simulink library "aeroblk_lib_HL20"  (Simulink 6.0)
settings: Solver=ode45  SolverMode=SingleTasking  StartTime=0.0  StopTime=10.0  RelTol=1e-3
values from neighbouring files (symbols this model uses):
  a_matrix = [-0.028840208852 -0.0156596305643 -0.0560912779756 -0.0863202941854 0.0209519994416 0.0112571762889 23.9049039727 0 2.90446405277 0 -10.5841662935 0 ... (11560 elements, 17x17x8x5)]    [aeroblk_HL20_autopilot_gains.mat]
  A_matrix = [-0.028840208852 -0.0156596305643 -0.0560912779756 -0.0863202941854 0.0209519994416 0.0112571762889 0 0 0 0 0 0 ... (11560 elements, 17x17x8x5)]    [aeroblk_HL20_autopilot_gains.mat]
  alpha_vec_Cn0 = [-10 -5 0 5 10 15 20 25 30]    [aeroblk_init_HL20.m]
  b_matrix = [-0.0157218860845 -0.283968320777 0.321370128412 0.271058535159 0.0185568065093 -0.00784369239396 -0.320886300542 1.82463546416 -0.0471251877299 0.142152392032 -0.0609086167769 0.505612659091 ... (2040 elements, 17x3x8x5)]    [aeroblk_HL20_autopilot_gains.mat]
  B_matrix = [0 0 0 0 0 0 4 0 0 0 0 0 ... (2040 elements, 17x3x8x5)]    [aeroblk_HL20_autopilot_gains.mat]
  b_ref = 13.89/m2ft    (= 4.23367186452)    [aeroblk_init_HL20.m]
  beta_vec_Cn0 = [0 2 5 10]    [aeroblk_init_HL20.m]
  c_matrix = [-5.97622599319 -0.726116013193 2.64604157338 -40.7494939461 11.661494324 21.0342779763 20.6745716213 -19.9416021106 -13.12545371 926.002157715 -187.969629212 -231.434488107 ... (2040 elements, 3x17x8x5)]    [aeroblk_HL20_autopilot_gains.mat]
  C_matrix = [0 0 0 0 0 0 0 0 0 -58.994812472 0 0 ... (2040 elements, 3x17x8x5)]    [aeroblk_HL20_autopilot_gains.mat]
  Clbeta = -0.00787    [aeroblk_init_HL20.m]
  Cm0 = reshape(temp(:,2),length(beta_vec_0),length(alpha_vec_0))    [aeroblk_init_HL20.m]
  CX0 = -reshape(temp(:,3),length(beta_vec_0),length(alpha_vec_0))    [aeroblk_init_HL20.m]
  CYbeta = -0.01242    [aeroblk_init_HL20.m]
  CZ0 = -reshape(temp(:,1),length(beta_vec_0),length(alpha_vec_0))    [aeroblk_init_HL20.m]
  d_matrix = [0 0 0 0 0 0 0 0 0 0 0 0 ... (360 elements, 3x3x8x5)]    [aeroblk_HL20_autopilot_gains.mat]
  d_ref = 0.75/m2ft    (= 0.228599992685)    [aeroblk_guid_dat.m]    (also in aeroblk_init_HL20.m = 8.60755172456)
  F_matrix = [5.97622599319 0.726116013193 -2.64604157338 40.7494939461 -11.661494324 -21.0342779763 -20.6745716213 19.9416021106 13.12545371 -926.002157715 187.969629212 231.434488107 ... (2040 elements, 3x17x8x5)]    [aeroblk_HL20_autopilot_gains.mat]
  H_matrix = [-0.0157218860845 -0.283968320777 0.321370128412 0.271058535159 0.0185568065093 -0.00784369239396 -0.320886300542 1.82463546416 -0.0471251877299 0.142152392032 -0.0609086167769 0.505612659091 ... (2040 elements, 17x3x8x5)]    [aeroblk_HL20_autopilot_gains.mat]
  mass = 13.98/Kg2slug    (= 204.022661401)    [aeroblk_guid_dat.m]    (also in aeroblk_init_HL20.m = 11738.9844962)
  x_cg = 0.575*len_veh    (= 4.78635044684)    [aeroblk_init_HL20.m]
  x_ref = 0.54*len_veh    (= 4.49500737616)    [aeroblk_init_HL20.m]
undefined symbols (not defined in the file or in its folder): F, Light, MIL
libraries: simulink x60, aerolibconvert x4, aerolibschedule x4, aerolibasang x3, aerolibwind2 x3, aeroblk_lib_HL20 x1, aerolib6dof2 x1, aerolibatmos2 x1, aerolibgravity2 x1, aerolibadyn x1
(part 1 of 2)
settings Model: Creator=The MathWorks Inc.  LastModifiedBy=batserve  ExtModeAutoUpdateStatusClock=off
settings OptimizationCC: BooleanDataType=off
settings DebuggingCC: CheckExecutionContextPreStartOutputMsg=on  CheckExecutionContextRuntimeOutputMsg=on  SolverPrmCheckMsg=none
settings HardwareCC: TargetUnknown=on

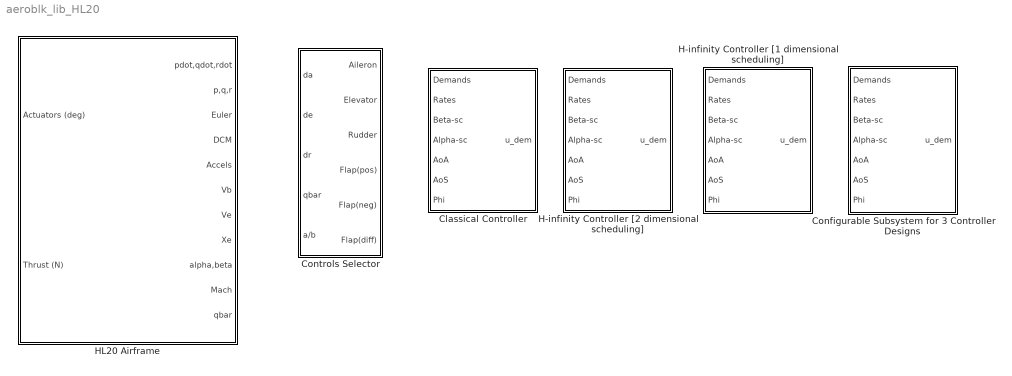
== system aeroblk_lib_HL20 ==
  Classical Controller : Subsystem  PropExecContextAcrossSSBoundary=on
  Configurable Subsystem for 3 Controller Designs : Subsystem  BlockChoice=Classical Controller  PropExecContextAcrossSSBoundary=on
      settings: TemplateBlock=self  MemberBlocks=Classical Controller,H-infinity Controller [1 dimensional scheduling],H-infinity Controller [2 dimensional scheduling]
  Controls Selector : Subsystem  PropExecContextAcrossSSBoundary=on
  H-infinity Controller [1 dimensional scheduling] : Subsystem  PropExecContextAcrossSSBoundary=on
  H-infinity Controller [2 dimensional scheduling] : Subsystem  PropExecContextAcrossSSBoundary=on
  HL20 Airframe : Subsystem  PropExecContextAcrossSSBoundary=on
      mask Display: image(imread('aeroblk_HL20pic.jpg','jpg'))

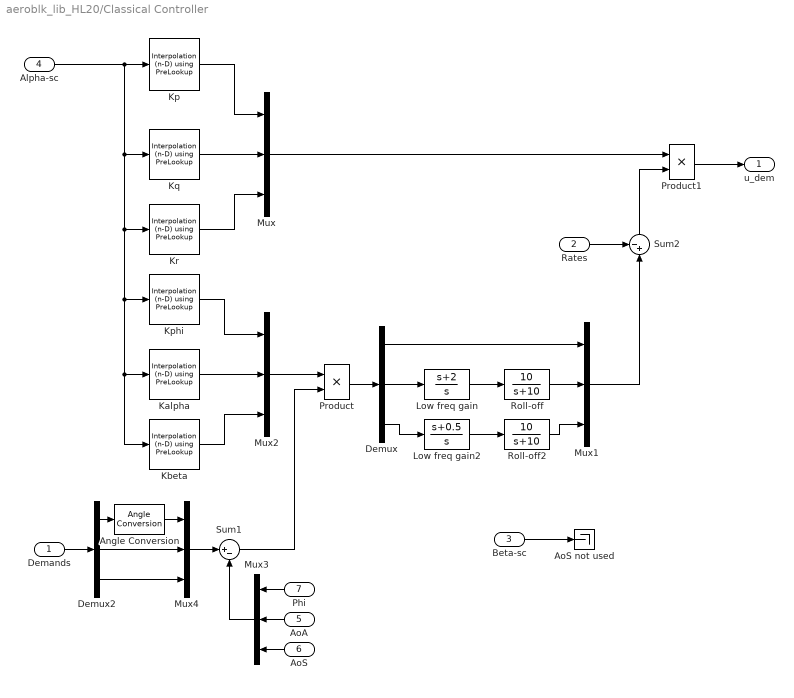
== system aeroblk_lib_HL20/Classical Controller ==
  Demands : Inport  Port=1  PortDimensions=3  LatchInput=off
  Rates : Inport  Port=2  PortDimensions=3  LatchInput=off
  Beta-sc : Inport  Port=3  LatchInput=off
  Alpha-sc : Inport  Port=4  LatchInput=off
  AoA : Inport  Orientation=left  Port=5  PortDimensions=1  LatchInput=off
  AoS : Inport  Orientation=left  Port=6  PortDimensions=1  LatchInput=off
  Phi : Inport  Orientation=left  Port=7  PortDimensions=1  LatchInput=off
  Angle Conversion : aerolibconvert/Angle Conversion  IU=deg  OU=rad
  AoS not used : Terminator
  Demux : Demux  Outputs=3
  Demux2 : Demux  Outputs=3
  Kalpha : simulink/Lookup Tables/Interpolation (n-D) using PreLookup  numDimsPopupSelect=1  explicitNumDims=2  table=Kalpha_1  interpMethod=Linear  extrapMethod=Linear  rangeErrorMode=None
  Kbeta : simulink/Lookup Tables/Interpolation (n-D) using PreLookup  numDimsPopupSelect=1  explicitNumDims=2  table=Kbeta_1  interpMethod=Linear  extrapMethod=Linear  rangeErrorMode=None
  Kp : simulink/Lookup Tables/Interpolation (n-D) using PreLookup  numDimsPopupSelect=1  explicitNumDims=2  table=Kp_1  interpMethod=Linear  extrapMethod=Linear  rangeErrorMode=None
  Kphi : simulink/Lookup Tables/Interpolation (n-D) using PreLookup  numDimsPopupSelect=1  explicitNumDims=2  table=Kphi_1  interpMethod=Linear  extrapMethod=Linear  rangeErrorMode=None
  Kq : simulink/Lookup Tables/Interpolation (n-D) using PreLookup  numDimsPopupSelect=1  explicitNumDims=2  table=Kq_1  interpMethod=Linear  extrapMethod=Linear  rangeErrorMode=None
  Kr : simulink/Lookup Tables/Interpolation (n-D) using PreLookup  numDimsPopupSelect=1  explicitNumDims=2  table=Kr_1  interpMethod=Linear  extrapMethod=Linear  rangeErrorMode=None
  Low freq gain : TransferFcn  Numerator=[1 2]  Denominator=[1 0]
  Low freq gain2 : TransferFcn  Numerator=[1 0.5]  Denominator=[1 0]
  Mux : Mux  Inputs=[1,1,1]
  Mux1 : Mux  Inputs=[1,1,1]
  Mux2 : Mux  Inputs=3
  Mux3 : Mux  Orientation=left  Inputs=[1,1,1]
  Mux4 : Mux  Inputs=[1,1,1]
  Product : Product  SaturateOnIntegerOverflow=on  InputSameDT=on
  Product1 : Product  SaturateOnIntegerOverflow=on  InputSameDT=on
  Roll-off : TransferFcn  Numerator=10  Denominator=[1 10]
  Roll-off2 : TransferFcn  Numerator=10  Denominator=[1 10]
  Sum1 : Sum  Inputs=|+-  SaturateOnIntegerOverflow=on  InputSameDT=on
  Sum2 : Sum  Orientation=up  Inputs=-+|  SaturateOnIntegerOverflow=on  InputSameDT=on
  u_dem : Outport  OutputWhenDisabled=reset  InitialOutput=[0 0 0]
  wires:
  Beta-sc/1 -> AoS not used/1
  Product1/1 -> u_dem/1
  Mux4/1 -> Sum1/1
  Demux2/3 -> Mux4/3
  Demux2/2 -> Mux4/2
  Angle Conversion/1 -> Mux4/1
  Demux2/1 -> Angle Conversion/1
  Demands/1 -> Demux2/1
  Kphi/1 -> Mux2/1
  Kbeta/1 -> Mux2/3
  Kalpha/1 -> Mux2/2
  Mux1/1 -> Sum2/2
  Sum2/1 -> Product1/2
  Mux/1 -> Product1/1
  Rates/1 -> Sum2/1
  Demux/1 -> Mux1/1
  Roll-off2/1 -> Mux1/3
  Roll-off/1 -> Mux1/2
  Demux/3 -> Low freq gain2/1
  Demux/2 -> Low freq gain/1
  Product/1 -> Demux/1
  Sum1/1 -> Product/2
  Mux2/1 -> Product/1
  AoS/1 -> Mux3/3
  AoA/1 -> Mux3/2
  Phi/1 -> Mux3/1
  Mux3/1 -> Sum1/2
  Low freq gain/1 -> Roll-off/1
  Low freq gain2/1 -> Roll-off2/1
  Kr/1 -> Mux/3
  Kp/1 -> Mux/1
  Kq/1 -> Mux/2
  Alpha-sc/1 -> Kbeta/1, Kalpha/1, Kphi/1, Kr/1, Kq/1, Kp/1

== system aeroblk_lib_HL20/Configurable Subsystem for 3 Controller Designs ==
  Demands : Inport  Port=1  LatchInput=off
  Rates : Inport  Port=2  LatchInput=off
  Beta-sc : Inport  Port=3  LatchInput=off
  Alpha-sc : Inport  Port=4  LatchInput=off
  AoA : Inport  Port=5  LatchInput=off
  AoS : Inport  Port=6  LatchInput=off
  Phi : Inport  Port=7  LatchInput=off
  Classical Controller : aeroblk_lib_HL20/Classical Controller  SimViewingDevice=off  DataTypeOverride=UseLocalSettings  MinMaxOverflowLogging=UseLocalSettings
      settings: Permissions=ReadWrite  RTWFcnNameOpts=Auto  RTWFileNameOpts=Auto
  u_dem : Outport
  wires:
  Demands/1 -> Classical Controller/1
  Rates/1 -> Classical Controller/2
  Beta-sc/1 -> Classical Controller/3
  Alpha-sc/1 -> Classical Controller/4
  AoA/1 -> Classical Controller/5
  AoS/1 -> Classical Controller/6
  Phi/1 -> Classical Controller/7
  Classical Controller/1 -> u_dem/1

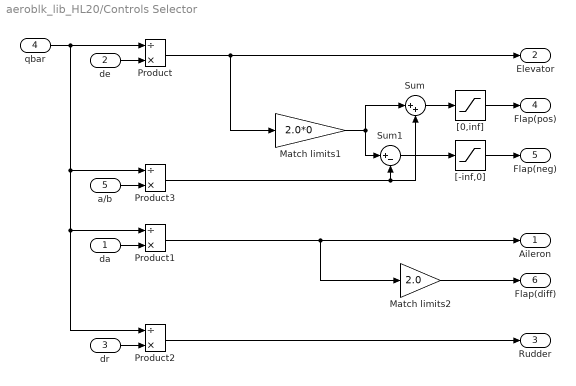
== system aeroblk_lib_HL20/Controls Selector ==
  da : Inport  Port=1  LatchInput=off
  de : Inport  Port=2  LatchInput=off
  dr : Inport  Port=3  LatchInput=off
  qbar : Inport  Port=4  LatchInput=off
  a/b : Inport  Port=5  LatchInput=off
  Match limits1 : Gain  Gain=2.0*0  SaturateOnIntegerOverflow=on
  Match limits2 : Gain  Gain=2.0  SaturateOnIntegerOverflow=on
  Product{,1..3} (4 alike) : Product  Inputs=/*  SaturateOnIntegerOverflow=on  InputSameDT=on
  Sum : Sum  Inputs=|++  SaturateOnIntegerOverflow=on  InputSameDT=on
  Sum1 : Sum  Inputs=|+-  SaturateOnIntegerOverflow=on  InputSameDT=on
  "[-inf,0]" : Saturate  UpperLimit=0  LowerLimit=-inf
  "[0,inf]" : Saturate  UpperLimit=inf  LowerLimit=0
  Aileron : Outport
  Elevator : Outport  Port=2
  Rudder : Outport  Port=3
  Flap(pos) : Outport  Port=4
  Flap(neg) : Outport  Port=5
  Flap(diff) : Outport  Port=6
  wires:
  qbar/1 -> Product/1, Product2/1, Product1/1, Product3/1
  de/1 -> Product/2
  Product2/1 -> Rudder/1
  dr/1 -> Product2/2
  da/1 -> Product1/2
  Product1/1 -> Match limits2/1, Aileron/1
  Product/1 -> Elevator/1, Match limits1/1
  Match limits1/1 -> Sum/1, Sum1/1
  "[-inf,0]"/1 -> Flap(neg)/1
  "[0,inf]"/1 -> Flap(pos)/1
  Match limits2/1 -> Flap(diff)/1
  a/b/1 -> Product3/2
  Sum/1 -> "[0,inf]"/1
  Sum1/1 -> "[-inf,0]"/1
  Product3/1 -> Sum1/2, Sum/2

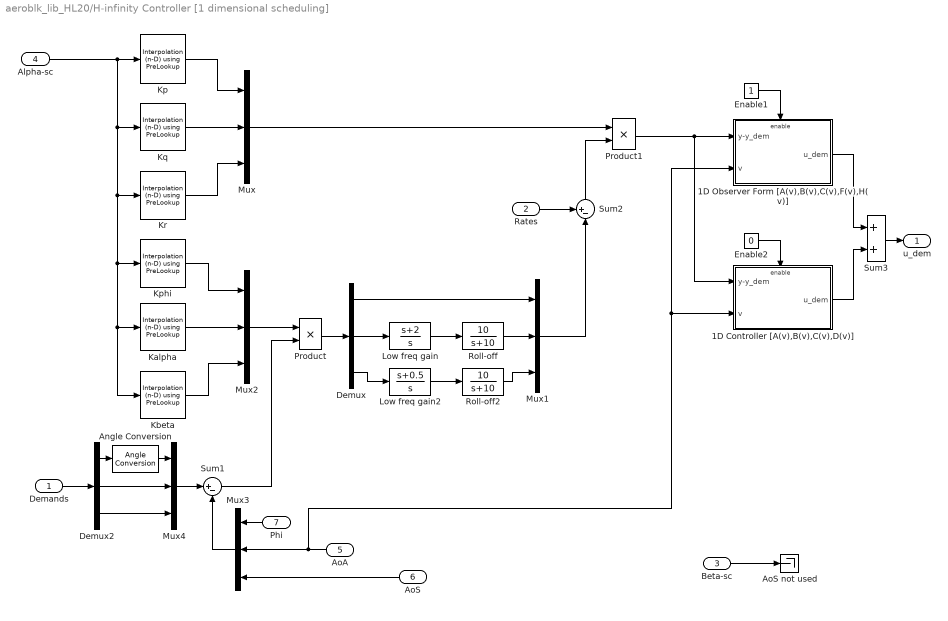
== system aeroblk_lib_HL20/H-infinity Controller [1 dimensional scheduling] ==
  Demands : Inport  Port=1  PortDimensions=3  LatchInput=off
  Rates : Inport  Port=2  PortDimensions=3  LatchInput=off
  Beta-sc : Inport  Port=3  LatchInput=off
  Alpha-sc : Inport  Port=4  LatchInput=off
  AoA : Inport  Orientation=left  Port=5  PortDimensions=1  LatchInput=off
  AoS : Inport  Orientation=left  Port=6  PortDimensions=1  LatchInput=off
  Phi : Inport  Orientation=left  Port=7  PortDimensions=1  LatchInput=off
  1D Controller [A(v),B(v),C(v),D(v)] : Subsystem  TreatAsAtomicUnit=on  PropExecContextAcrossSSBoundary=on
  1D Observer Form [A(v),B(v),C(v),F(v),H(v)] : Subsystem  TreatAsAtomicUnit=on  PropExecContextAcrossSSBoundary=on
  Angle Conversion : aerolibconvert/Angle Conversion  IU=deg  OU=rad
  AoS not used : Terminator
  Demux : Demux  Outputs=3
  Demux2 : Demux  Outputs=3
  Enable1 : Constant
  Enable2 : Constant  Value=0
  Kalpha : simulink/Lookup Tables/Interpolation (n-D) using PreLookup  numDimsPopupSelect=1  explicitNumDims=2  table=Kalpha_1  interpMethod=Linear  extrapMethod=Linear  rangeErrorMode=None
  Kbeta : simulink/Lookup Tables/Interpolation (n-D) using PreLookup  numDimsPopupSelect=1  explicitNumDims=2  table=Kbeta_1  interpMethod=Linear  extrapMethod=Linear  rangeErrorMode=None
  Kp : simulink/Lookup Tables/Interpolation (n-D) using PreLookup  numDimsPopupSelect=1  explicitNumDims=2  table=Kp_1  interpMethod=Linear  extrapMethod=Linear  rangeErrorMode=None
  Kphi : simulink/Lookup Tables/Interpolation (n-D) using PreLookup  numDimsPopupSelect=1  explicitNumDims=2  table=Kphi_1  interpMethod=Linear  extrapMethod=Linear  rangeErrorMode=None
  Kq : simulink/Lookup Tables/Interpolation (n-D) using PreLookup  numDimsPopupSelect=1  explicitNumDims=2  table=Kq_1  interpMethod=Linear  extrapMethod=Linear  rangeErrorMode=None
  Kr : simulink/Lookup Tables/Interpolation (n-D) using PreLookup  numDimsPopupSelect=1  explicitNumDims=2  table=Kr_1  interpMethod=Linear  extrapMethod=Linear  rangeErrorMode=None
  Low freq gain : TransferFcn  Numerator=[1 2]  Denominator=[1 0]
  Low freq gain2 : TransferFcn  Numerator=[1 0.5]  Denominator=[1 0]
  Mux : Mux  Inputs=[1,1,1]
  Mux1 : Mux  Inputs=[1,1,1]
  Mux2 : Mux  Inputs=3
  Mux3 : Mux  Orientation=left  Inputs=[1,1,1]
  Mux4 : Mux  Inputs=[1,1,1]
  Product : Product  SaturateOnIntegerOverflow=on  InputSameDT=on
  Product1 : Product  SaturateOnIntegerOverflow=on  InputSameDT=on
  Roll-off : TransferFcn  Numerator=10  Denominator=[1 10]
  Roll-off2 : TransferFcn  Numerator=10  Denominator=[1 10]
  Sum1 : Sum  Inputs=|+-  SaturateOnIntegerOverflow=on  InputSameDT=on
  Sum2 : Sum  Orientation=up  Inputs=+-|  SaturateOnIntegerOverflow=on  InputSameDT=on
  Sum3 : Sum  SaturateOnIntegerOverflow=on  InputSameDT=on
  u_dem : Outport  OutputWhenDisabled=reset  InitialOutput=[0 0 0]
  wires:
  Beta-sc/1 -> AoS not used/1
  Mux4/1 -> Sum1/1
  Demux2/3 -> Mux4/3
  Demux2/2 -> Mux4/2
  Angle Conversion/1 -> Mux4/1
  Demux2/1 -> Angle Conversion/1
  Demands/1 -> Demux2/1
  Kphi/1 -> Mux2/1
  Kbeta/1 -> Mux2/3
  Kalpha/1 -> Mux2/2
  Mux1/1 -> Sum2/2
  Sum2/1 -> Product1/2
  Mux/1 -> Product1/1
  Rates/1 -> Sum2/1
  Demux/1 -> Mux1/1
  Roll-off2/1 -> Mux1/3
  Roll-off/1 -> Mux1/2
  Demux/3 -> Low freq gain2/1
  Demux/2 -> Low freq gain/1
  Product/1 -> Demux/1
  Sum1/1 -> Product/2
  Mux2/1 -> Product/1
  AoS/1 -> Mux3/3
  AoA/1 -> 1D Observer Form [A(v),B(v),C(v),F(v),H(v)]/2(v), 1D Controller [A(v),B(v),C(v),D(v)]/2(v), Mux3/2
  Phi/1 -> Mux3/1
  Mux3/1 -> Sum1/2
  Low freq gain/1 -> Roll-off/1
  Low freq gain2/1 -> Roll-off2/1
  Kr/1 -> Mux/3
  Kp/1 -> Mux/1
  Kq/1 -> Mux/2
  Alpha-sc/1 -> Kbeta/1, Kalpha/1, Kphi/1, Kr/1, Kq/1, Kp/1
  Product1/1 -> 1D Observer Form [A(v),B(v),C(v),F(v),H(v)]/1(y-y_dem), 1D Controller [A(v),B(v),C(v),D(v)]/1(y-y_dem)
  Enable1/1 -> 1D Observer Form [A(v),B(v),C(v),F(v),H(v)]/Enable
  Enable2/1 -> 1D Controller [A(v),B(v),C(v),D(v)]/Enable
  1D Observer Form [A(v),B(v),C(v),F(v),H(v)]/1(u_dem) -> Sum3/1
  1D Controller [A(v),B(v),C(v),D(v)]/1(u_dem) -> Sum3/2
  Sum3/1 -> u_dem/1

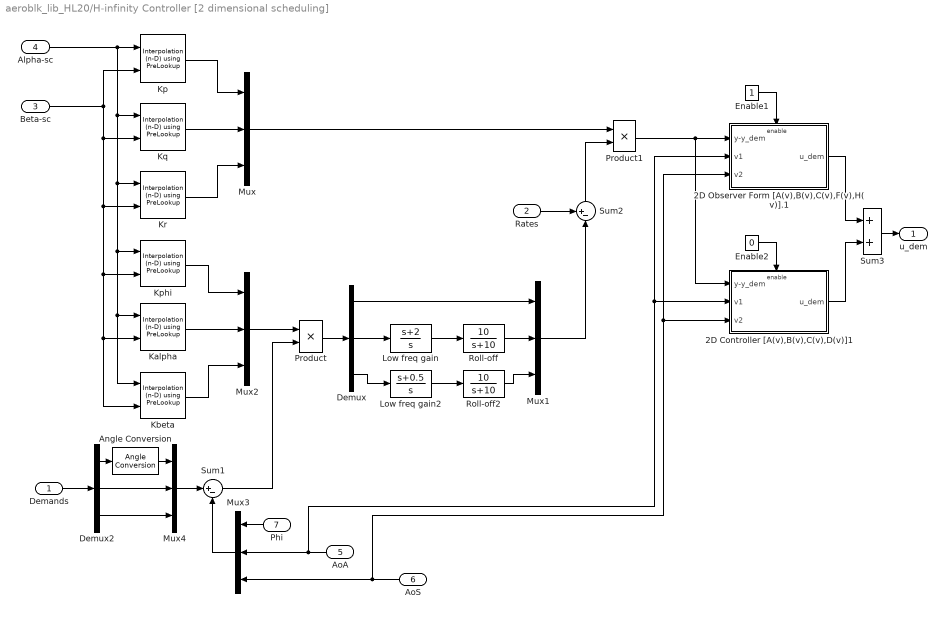
== system aeroblk_lib_HL20/H-infinity Controller [2 dimensional scheduling] ==
  Demands : Inport  Port=1  PortDimensions=3  LatchInput=off
  Rates : Inport  Port=2  PortDimensions=3  LatchInput=off
  Beta-sc : Inport  Port=3  LatchInput=off
  Alpha-sc : Inport  Port=4  LatchInput=off
  AoA : Inport  Orientation=left  Port=5  PortDimensions=1  LatchInput=off
  AoS : Inport  Orientation=left  Port=6  PortDimensions=1  LatchInput=off
  Phi : Inport  Orientation=left  Port=7  PortDimensions=1  LatchInput=off
  2D Controller [A(v),B(v),C(v),D(v)]1 : Subsystem  TreatAsAtomicUnit=on  PropExecContextAcrossSSBoundary=on
  2D Observer Form [A(v),B(v),C(v),F(v),H(v)].1 : Subsystem  TreatAsAtomicUnit=on  PropExecContextAcrossSSBoundary=on
  Angle Conversion : aerolibconvert/Angle Conversion  IU=deg  OU=rad
  Demux : Demux  Outputs=3
  Demux2 : Demux  Outputs=3
  Enable1 : Constant
  Enable2 : Constant  Value=0
  Kalpha : simulink/Lookup Tables/Interpolation (n-D) using PreLookup  numDimsPopupSelect=2  explicitNumDims=2  table=Kalpha  interpMethod=Linear  extrapMethod=Linear  rangeErrorMode=None
  Kbeta : simulink/Lookup Tables/Interpolation (n-D) using PreLookup  numDimsPopupSelect=2  explicitNumDims=2  table=Kbeta  interpMethod=Linear  extrapMethod=Linear  rangeErrorMode=None
  Kp : simulink/Lookup Tables/Interpolation (n-D) using PreLookup  numDimsPopupSelect=2  explicitNumDims=2  table=Kp  interpMethod=Linear  extrapMethod=Linear  rangeErrorMode=None
  Kphi : simulink/Lookup Tables/Interpolation (n-D) using PreLookup  numDimsPopupSelect=2  explicitNumDims=2  table=Kphi  interpMethod=Linear  extrapMethod=Linear  rangeErrorMode=None
  Kq : simulink/Lookup Tables/Interpolation (n-D) using PreLookup  numDimsPopupSelect=2  explicitNumDims=2  table=Kq  interpMethod=Linear  extrapMethod=Linear  rangeErrorMode=None
  Kr : simulink/Lookup Tables/Interpolation (n-D) using PreLookup  numDimsPopupSelect=2  explicitNumDims=2  table=Kr  interpMethod=Linear  extrapMethod=Linear  rangeErrorMode=None
  Low freq gain : TransferFcn  Numerator=[1 2]  Denominator=[1 0]
  Low freq gain2 : TransferFcn  Numerator=[1 0.5]  Denominator=[1 0]
  Mux : Mux  Inputs=[1,1,1]
  Mux1 : Mux  Inputs=[1,1,1]
  Mux2 : Mux  Inputs=3
  Mux3 : Mux  Orientation=left  Inputs=[1,1,1]
  Mux4 : Mux  Inputs=[1,1,1]
  Product : Product  SaturateOnIntegerOverflow=on  InputSameDT=on
  Product1 : Product  SaturateOnIntegerOverflow=on  InputSameDT=on
  Roll-off : TransferFcn  Numerator=10  Denominator=[1 10]
  Roll-off2 : TransferFcn  Numerator=10  Denominator=[1 10]
  Sum1 : Sum  Inputs=|+-  SaturateOnIntegerOverflow=on  InputSameDT=on
  Sum2 : Sum  Orientation=up  Inputs=+-|  SaturateOnIntegerOverflow=on  InputSameDT=on
  Sum3 : Sum  SaturateOnIntegerOverflow=on  InputSameDT=on
  u_dem : Outport  OutputWhenDisabled=reset  InitialOutput=[0 0 0]
  wires:
  Sum3/1 -> u_dem/1
  2D Controller [A(v),B(v),C(v),D(v)]1/1(u_dem) -> Sum3/2
  2D Observer Form [A(v),B(v),C(v),F(v),H(v)].1/1(u_dem) -> Sum3/1
  Enable2/1 -> 2D Controller [A(v),B(v),C(v),D(v)]1/Enable
  Enable1/1 -> 2D Observer Form [A(v),B(v),C(v),F(v),H(v)].1/Enable
  Product1/1 -> 2D Observer Form [A(v),B(v),C(v),F(v),H(v)].1/1(y-y_dem), 2D Controller [A(v),B(v),C(v),D(v)]1/1(y-y_dem)
  Beta-sc/1 -> Kp/2, Kalpha/2, Kbeta/2, Kphi/2, Kr/2, Kq/2
  Alpha-sc/1 -> Kp/1, Kq/1, Kr/1, Kphi/1, Kalpha/1, Kbeta/1
  Kq/1 -> Mux/2
  Kp/1 -> Mux/1
  Kr/1 -> Mux/3
  Low freq gain2/1 -> Roll-off2/1
  Low freq gain/1 -> Roll-off/1
  Mux3/1 -> Sum1/2
  Phi/1 -> Mux3/1
  AoA/1 -> 2D Observer Form [A(v),B(v),C(v),F(v),H(v)].1/2(v1), 2D Controller [A(v),B(v),C(v),D(v)]1/2(v1), Mux3/2
  AoS/1 -> 2D Observer Form [A(v),B(v),C(v),F(v),H(v)].1/3(v2), 2D Controller [A(v),B(v),C(v),D(v)]1/3(v2), Mux3/3
  Mux2/1 -> Product/1
  Sum1/1 -> Product/2
  Product/1 -> Demux/1
  Demux/2 -> Low freq gain/1
  Demux/3 -> Low freq gain2/1
  Roll-off/1 -> Mux1/2
  Roll-off2/1 -> Mux1/3
  Demux/1 -> Mux1/1
  Rates/1 -> Sum2/1
  Mux/1 -> Product1/1
  Sum2/1 -> Product1/2
  Mux1/1 -> Sum2/2
  Kalpha/1 -> Mux2/2
  Kbeta/1 -> Mux2/3
  Kphi/1 -> Mux2/1
  Demands/1 -> Demux2/1
  Demux2/1 -> Angle Conversion/1
  Angle Conversion/1 -> Mux4/1
  Demux2/2 -> Mux4/2
  Demux2/3 -> Mux4/3
  Mux4/1 -> Sum1/1

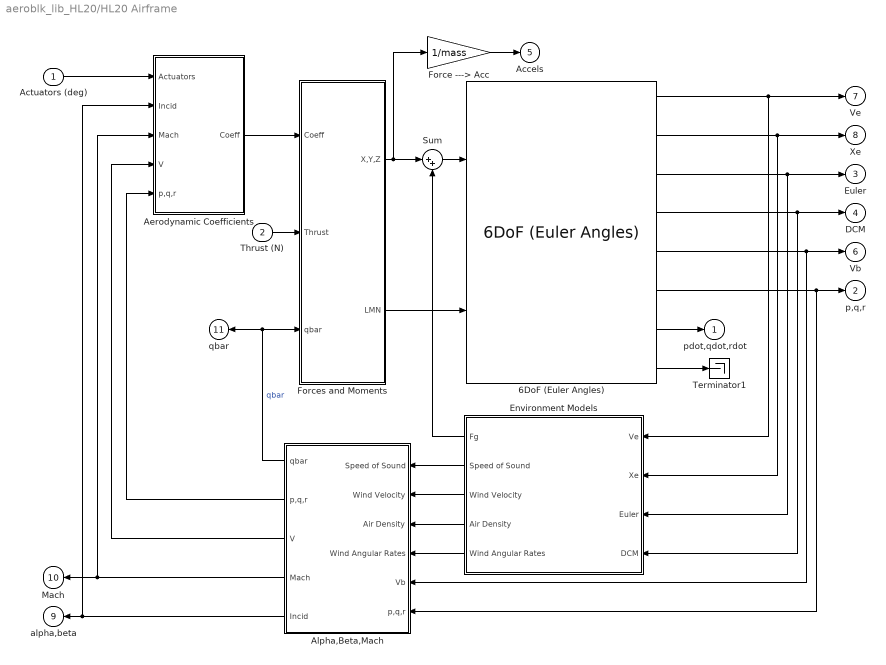
== system aeroblk_lib_HL20/HL20 Airframe ==
  Actuators (deg) : Inport  Port=1  LatchInput=off
  Thrust (N) : Inport  Port=2  LatchInput=off
  6DoF (Euler Angles) : aerolib6dof2/6DoF (Euler Angles)  units=Metric (MKS)  mtype=Fixed  rep=Euler Angles  xme_0=xme_0  Vm_0=Vmw  eul_0=Euler_0  pm_0=pm_0  mass_0=mass  mass_e=0.5  mass_f=2.0  inertia=Inertia  inertia_e=eye(3)  inertia_f=2*eye(3)  k_quat=1.0
  Aerodynamic Coefficients : Subsystem  PropExecContextAcrossSSBoundary=on
  Alpha,Beta,Mach : Subsystem  Orientation=left  PropExecContextAcrossSSBoundary=on
  Environment Models : Subsystem  Orientation=left  PropExecContextAcrossSSBoundary=on
  Force ---> Acc : Gain  Gain=1/mass  SaturateOnIntegerOverflow=on
  Forces and Moments : Subsystem  PropExecContextAcrossSSBoundary=on
  Sum : Sum  Inputs=|++  SaturateOnIntegerOverflow=on  InputSameDT=on
  Terminator1 : Terminator
  pdot,qdot,rdot : Outport  InitialOutput=0
  p,q,r : Outport  Port=2  InitialOutput=0
  Euler : Outport  Port=3  InitialOutput=0
  DCM : Outport  Port=4  InitialOutput=0
  Accels : Outport  Port=5  InitialOutput=0
  Vb : Outport  Port=6  InitialOutput=0
  Ve : Outport  Port=7  InitialOutput=0
  Xe : Outport  Port=8  InitialOutput=0
  alpha,beta : Outport  Orientation=left  Port=9  InitialOutput=0
  Mach : Outport  Orientation=left  Port=10  InitialOutput=0
  qbar : Outport  Orientation=left  Port=11  InitialOutput=0
  wires:
  Environment Models/5(Wind Angular Rates) -> Alpha,Beta,Mach/4(Wind Angular Rates)
  Alpha,Beta,Mach/2("p,q,r ") -> Aerodynamic Coefficients/5(p,q,r)
  Alpha,Beta,Mach/4(Mach) -> Mach/1, Aerodynamic Coefficients/3(Mach)
  Alpha,Beta,Mach/3(V) -> Aerodynamic Coefficients/4(V)
  Actuators (deg)/1 -> Aerodynamic Coefficients/1(Actuators)
  Force ---> Acc/1 -> Accels/1
  Environment Models/1(Fg) -> Sum/2
  Sum/1 -> 6DoF (Euler Angles)/1
  Forces and Moments/1(X,Y,Z) -> Sum/1, Force ---> Acc/1
  Alpha,Beta,Mach/1(qbar) -> qbar/1, Forces and Moments/3(qbar)  "qbar"
  Forces and Moments/2(LMN) -> 6DoF (Euler Angles)/2
  Environment Models/4(Air Density) -> Alpha,Beta,Mach/3(Air Density)
  Environment Models/2(Speed of Sound) -> Alpha,Beta,Mach/1(Speed of Sound)
  6DoF (Euler Angles)/5 -> Vb/1, Alpha,Beta,Mach/5(Vb)
  Environment Models/3(Wind Velocity) -> Alpha,Beta,Mach/2(Wind Velocity)
  Aerodynamic Coefficients/1(Coeff) -> Forces and Moments/1(Coeff)
  Alpha,Beta,Mach/5(Incid) -> Aerodynamic Coefficients/2(Incid), alpha,beta/1
  6DoF (Euler Angles)/3 -> Euler/1, Environment Models/3(Euler)
  6DoF (Euler Angles)/4 -> Environment Models/4(DCM), DCM/1
  6DoF (Euler Angles)/7 -> pdot,qdot,rdot/1
  Thrust (N)/1 -> Forces and Moments/2(Thrust)
  6DoF (Euler Angles)/6 -> Alpha,Beta,Mach/6(p,q,r), p,q,r/1
  6DoF (Euler Angles)/2 -> Xe/1, Environment Models/2(Xe)
  6DoF (Euler Angles)/1 -> Ve/1, Environment Models/1(Ve)
  6DoF (Euler Angles)/8 -> Terminator1/1

== system aeroblk_lib_HL20/H-infinity Controller [1 dimensional scheduling]/1D Controller [A(v),B(v),C(v),D(v)] ==
  y-y_dem : Inport  Port=1  PortDimensions=3  LatchInput=off
  v : Inport  Port=2  PortDimensions=1  LatchInput=off
  Enable : EnablePort
  -1 : Gain  Gain=-1  SaturateOnIntegerOverflow=on
  1D Controller [A(v),B(v),C(v),D(v)] : aerolibschedule/1D Controller [A(v),B(v),C(v),D(v)]  A=squeeze(a_matrix(:,:,:,3))  B=squeeze(b_matrix(:,:,:,3))  C=squeeze(c_matrix(:,:,:,3))  D=squeeze(d_matrix(:,:,:,3))  AoA_vec=a_vec  x_initial=0
  u_dem : Outport  OutputWhenDisabled=reset  InitialOutput=[0 0 0]
  wires:
  y-y_dem/1 -> -1/1
  -1/1 -> 1D Controller [A(v),B(v),C(v),D(v)]/1
  1D Controller [A(v),B(v),C(v),D(v)]/1 -> u_dem/1
  v/1 -> 1D Controller [A(v),B(v),C(v),D(v)]/2

== system aeroblk_lib_HL20/H-infinity Controller [1 dimensional scheduling]/1D Observer Form [A(v),B(v),C(v),F(v),H(v)] ==
  y-y_dem : Inport  Port=1  PortDimensions=3  LatchInput=off
  v : Inport  Port=2  PortDimensions=1  LatchInput=off
  Enable : EnablePort
  1D Observer Form [A(v),B(v),C(v),F(v),H(v)] : aerolibschedule/1D Observer Form [A(v),B(v),C(v),F(v),H(v)]  A=squeeze(A_matrix(:,:,:,3))  B=squeeze(B_matrix(:,:,:,3))  C=squeeze(C_matrix(:,:,:,3))  F=squeeze(F_matrix(:,:,:,3))  H=squeeze(H_matrix(:,:,:,3))  AoA_vec=a_vec  x_initial=0
  Signal Specification : simulink/Signal Attributes/Signal Specification  D=3  Ts=-1  DataType=auto  OutDataType=sfix(16)  OutScaling=2^0
      settings: SignalType=auto  SamplingMode=auto
  u_dem : Outport  OutputWhenDisabled=reset  InitialOutput=[0 0 0]
  wires:
  y-y_dem/1 -> 1D Observer Form [A(v),B(v),C(v),F(v),H(v)]/1
  v/1 -> 1D Observer Form [A(v),B(v),C(v),F(v),H(v)]/2
  1D Observer Form [A(v),B(v),C(v),F(v),H(v)]/1 -> Signal Specification/1
  Signal Specification/1 -> 1D Observer Form [A(v),B(v),C(v),F(v),H(v)]/3, u_dem/1

== system aeroblk_lib_HL20/H-infinity Controller [2 dimensional scheduling]/2D Controller [A(v),B(v),C(v),D(v)]1 ==
  y-y_dem : Inport  Port=1  PortDimensions=3  LatchInput=off
  v1 : Inport  Port=2  PortDimensions=1  LatchInput=off
  v2 : Inport  Port=3  PortDimensions=1  LatchInput=off
  Enable : EnablePort
  -1 : Gain  Gain=-1  SaturateOnIntegerOverflow=on
  2D Controller [A(v),B(v),C(v),D(v)]1 : aerolibschedule/2D Controller [A(v),B(v),C(v),D(v)]  A=a_matrix  B=b_matrix  C=c_matrix  D=d_matrix  AoA_vec=a_vec  Mach_vec=b_vec  x_initial=0
  u_dem : Outport  OutputWhenDisabled=reset  InitialOutput=[0 0 0]
  wires:
  v2/1 -> 2D Controller [A(v),B(v),C(v),D(v)]1/3
  v1/1 -> 2D Controller [A(v),B(v),C(v),D(v)]1/2
  2D Controller [A(v),B(v),C(v),D(v)]1/1 -> u_dem/1
  -1/1 -> 2D Controller [A(v),B(v),C(v),D(v)]1/1
  y-y_dem/1 -> -1/1

== system aeroblk_lib_HL20/H-infinity Controller [2 dimensional scheduling]/2D Observer Form [A(v),B(v),C(v),F(v),H(v)].1 ==
  y-y_dem : Inport  Port=1  PortDimensions=3  LatchInput=off
  v1 : Inport  Port=2  PortDimensions=1  LatchInput=off
  v2 : Inport  Port=3  PortDimensions=1  LatchInput=off
  Enable : EnablePort
  2D Observer Form [A(v),B(v),C(v),F(v),H(v)] : aerolibschedule/2D Observer Form [A(v),B(v),C(v),F(v),H(v)]  A=A_matrix  B=B_matrix  C=C_matrix  F=F_matrix  H=H_matrix  AoA_vec=a_vec  Mach_vec=b_vec  x_initial=0
  Signal Specification : simulink/Signal Attributes/Signal Specification  D=3  Ts=-1  DataType=auto  OutDataType=sfix(16)  OutScaling=2^0
      settings: SignalType=auto  SamplingMode=auto
  u_dem : Outport  OutputWhenDisabled=reset  InitialOutput=[0 0 0]
  wires:
  Signal Specification/1 -> 2D Observer Form [A(v),B(v),C(v),F(v),H(v)]/4, u_dem/1
  2D Observer Form [A(v),B(v),C(v),F(v),H(v)]/1 -> Signal Specification/1
  v2/1 -> 2D Observer Form [A(v),B(v),C(v),F(v),H(v)]/3
  v1/1 -> 2D Observer Form [A(v),B(v),C(v),F(v),H(v)]/2
  y-y_dem/1 -> 2D Observer Form [A(v),B(v),C(v),F(v),H(v)]/1

== system aeroblk_lib_HL20/HL20 Airframe/Aerodynamic Coefficients ==
  Actuators : Inport  Port=1  LatchInput=off
  Incid : Inport  Port=2  LatchInput=off
  Mach : Inport  Port=3  LatchInput=off
  V : Inport  Port=4  LatchInput=off
  p,q,r : Inport  Port=5  LatchInput=off
  Actuator Increments : Subsystem  PropExecContextAcrossSSBoundary=on
  Angle Conversion : aerolibconvert/Angle Conversion  IU=rad  OU=deg
  Body Rate Damping : Subsystem  PropExecContextAcrossSSBoundary=on
  Datum Coefficients : Subsystem  PropExecContextAcrossSSBoundary=on
  Demux : Demux  Outputs=2
  Sum1 : Sum  Inputs=+++  SaturateOnIntegerOverflow=on  InputSameDT=on
  Terminator2 : Terminator
  Coeff : Outport  InitialOutput=0
  wires:
  Demux/1 -> Datum Coefficients/1(Alpha), Actuator Increments/1(Alpha), Body Rate Damping/3(Alpha)
  p,q,r/1 -> Body Rate Damping/2(p,q,r)
  Incid/1 -> Angle Conversion/1
  Angle Conversion/1 -> Demux/1
  Actuators/1 -> Actuator Increments/3("Actuator Deflections ")
  Sum1/1 -> Coeff/1
  Datum Coefficients/1(cl) -> Sum1/2
  Demux/2 -> Datum Coefficients/2(Beta), Actuator Increments/2(Beta)
  Mach/1 -> Terminator2/1
  V/1 -> Body Rate Damping/1(V)
  Body Rate Damping/1(cl) -> Sum1/1
  Actuator Increments/1(cl) -> Sum1/3

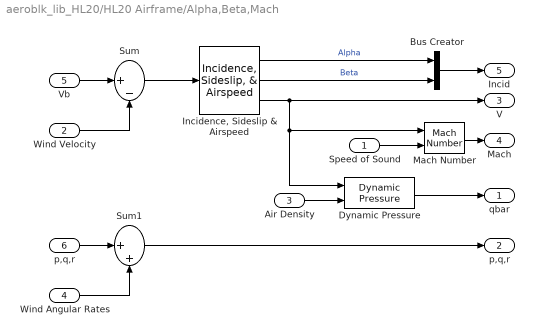
== system aeroblk_lib_HL20/HL20 Airframe/Alpha,Beta,Mach ==
  Speed of Sound : Inport  Port=1  LatchInput=off
  Wind Velocity : Inport  Port=2  PortDimensions=3  LatchInput=off
  Air Density : Inport  Port=3  LatchInput=off
  Wind Angular Rates : Inport  Port=4  PortDimensions=3  LatchInput=off
  Vb : Inport  Port=5  PortDimensions=3  LatchInput=off
  p,q,r : Inport  Port=6  PortDimensions=3  LatchInput=off
  Bus Creator : BusCreator  DialogController=Simulink.DDGSource_Bus  Inputs=2
  Dynamic Pressure : aerolibasang/Dynamic Pressure
  "Incidence, Sideslip & Airspeed" : aerolibasang/Incidence, Sideslip, & Airspeed
  Mach Number : aerolibasang/Mach Number
  Sum : Sum  Inputs=|+-  SaturateOnIntegerOverflow=on  InputSameDT=on
  Sum1 : Sum  Inputs=|++  SaturateOnIntegerOverflow=on  InputSameDT=on
  qbar : Outport  InitialOutput=0
  "p,q,r " : Outport  Port=2
  V : Outport  Port=3
  Mach : Outport  Port=4
  Incid : Outport  Port=5
  wires:
  Sum1/1 -> "p,q,r "/1
  Wind Angular Rates/1 -> Sum1/2
  p,q,r/1 -> Sum1/1
  "Incidence, Sideslip & Airspeed"/1 -> Bus Creator/1  "Alpha"
  Bus Creator/1 -> Incid/1
  "Incidence, Sideslip & Airspeed"/2 -> Bus Creator/2  "Beta"
  Wind Velocity/1 -> Sum/2
  Speed of Sound/1 -> Mach Number/2
  Vb/1 -> Sum/1
  Sum/1 -> "Incidence, Sideslip & Airspeed"/1
  "Incidence, Sideslip & Airspeed"/3 -> V/1, Dynamic Pressure/1, Mach Number/1
  Mach Number/1 -> Mach/1
  Air Density/1 -> Dynamic Pressure/2
  Dynamic Pressure/1 -> qbar/1

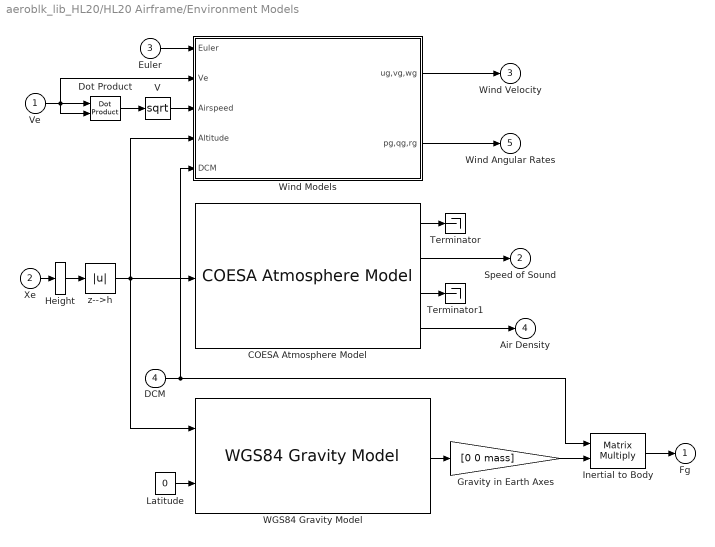
== system aeroblk_lib_HL20/HL20 Airframe/Environment Models ==
  Ve : Inport  Port=1  LatchInput=off
  Xe : Inport  Port=2  PortDimensions=3  LatchInput=off
  Euler : Inport  Port=3  LatchInput=off
  DCM : Inport  Port=4  LatchInput=off
  COESA Atmosphere Model : aerolibatmos2/COESA Atmosphere Model  units=Metric (MKS)  spec=1976 COESA-extended U.S. Standard Atmosphere  model=Profile  profile_var=High temperature  profile_percent=10%  profile_alt=5 km (16404 ft)  envelope_var=High temperature  envelope_percent=1%  action=None
  Dot Product : simulink/Math Operations/Dot Product  OutDataType=sfix(16)  OutScaling=2^-10  DoSatur=on
  Gravity in Earth Axes : Gain  Gain=[0 0 mass]  SaturateOnIntegerOverflow=on
  Height : Selector  Elements=[3]  InputPortWidth=3
  Inertial to Body : Product  Multiplication=Matrix(*)  SaturateOnIntegerOverflow=on  InputSameDT=on
  Latitude : Constant  Value=0
  Terminator : Terminator
  Terminator1 : Terminator
  V : Math  Operator=sqrt  SaturateOnIntegerOverflow=on
  WGS84 Gravity Model : aerolibgravity2/WGS84 Gravity Model  model=WGS84 Taylor Series  units=Metric (MKS)  no_atmos=on  precessing=on  month=February  day=1  year=2000  no_centrifugal=on  action=None
  Wind Models : Subsystem  PropExecContextAcrossSSBoundary=on
  z-->h : Abs  SaturateOnIntegerOverflow=on
  Fg : Outport  InitialOutput=0
  Speed of Sound : Outport  Port=2  InitialOutput=0
  Wind Velocity : Outport  Port=3  InitialOutput=0
  Air Density : Outport  Port=4  InitialOutput=0
  Wind Angular Rates : Outport  Port=5  InitialOutput=0
  wires:
  V/1 -> Wind Models/3(Airspeed)
  Inertial to Body/1 -> Fg/1
  DCM/1 -> Inertial to Body/1, Wind Models/5(DCM)
  Gravity in Earth Axes/1 -> Inertial to Body/2
  WGS84 Gravity Model/1 -> Gravity in Earth Axes/1
  Latitude/1 -> WGS84 Gravity Model/2
  Xe/1 -> Height/1
  Height/1 -> z-->h/1
  COESA Atmosphere Model/1 -> Terminator/1
  COESA Atmosphere Model/3 -> Terminator1/1
  COESA Atmosphere Model/2 -> Speed of Sound/1
  COESA Atmosphere Model/4 -> Air Density/1
  z-->h/1 -> Wind Models/4(Altitude), WGS84 Gravity Model/1, COESA Atmosphere Model/1
  Dot Product/1 -> V/1
  Wind Models/2(pg,qg,rg) -> Wind Angular Rates/1
  Wind Models/1(ug,vg,wg) -> Wind Velocity/1
  Ve/1 -> Dot Product/2, Dot Product/1, Wind Models/2(Ve)
  Euler/1 -> Wind Models/1(Euler)

== system aeroblk_lib_HL20/HL20 Airframe/Forces and Moments ==
  Coeff : Inport  Port=1  LatchInput=off
  Thrust : Inport  Orientation=down  Port=2  LatchInput=off
  qbar : Inport  Port=3  LatchInput=off
  Aerodynamic Forces and Moments : aerolibadyn/Aerodynamic Forces and Moments  S=S_ref  b=b_ref  cbar=d_ref
  Center of Gravity : Constant  Value=[-x_cg 0 0]
  Center of Pressure : Constant  Value=[- x_ref 0 0]
  Sum : Sum  Inputs=++|  SaturateOnIntegerOverflow=on  InputSameDT=on
  X,Y,Z : Outport  InitialOutput=0
  LMN : Outport  Port=2  InitialOutput=0
  wires:
  Coeff/1 -> Aerodynamic Forces and Moments/1
  qbar/1 -> Aerodynamic Forces and Moments/2
  Thrust/1 -> Sum/1
  Sum/1 -> X,Y,Z/1
  Aerodynamic Forces and Moments/2 -> LMN/1
  Aerodynamic Forces and Moments/1 -> Sum/2
  Center of Gravity/1 -> Aerodynamic Forces and Moments/3
  Center of Pressure/1 -> Aerodynamic Forces and Moments/4

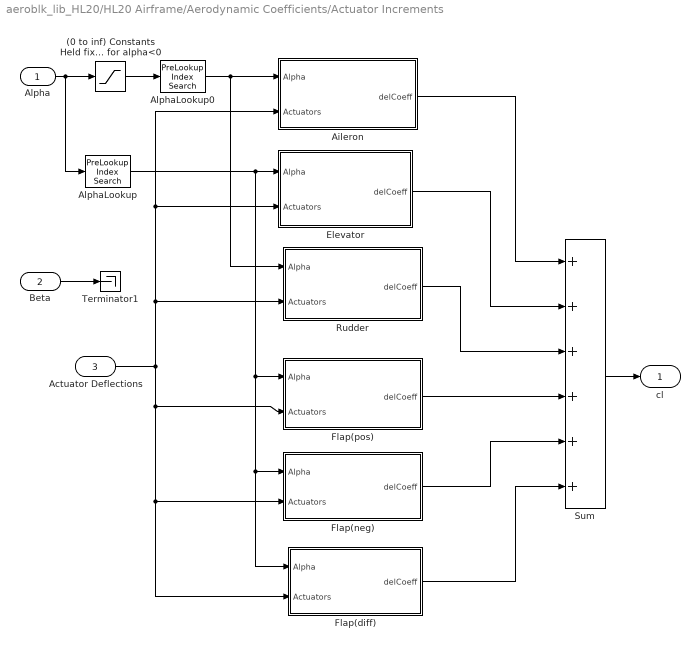
== system aeroblk_lib_HL20/HL20 Airframe/Aerodynamic Coefficients/Actuator Increments ==
  Alpha : Inport  Port=1  LatchInput=off
  Beta : Inport  Port=2  LatchInput=off
  "Actuator Deflections " : Inport  Port=3  LatchInput=off
  (0 to inf) Constants Held fixed for alpha<0 : Saturate  UpperLimit=inf  LowerLimit=0
  Aileron : Subsystem  PropExecContextAcrossSSBoundary=on
  AlphaLookup : simulink/Lookup Tables/PreLookup Index Search  bpData=alpha_vec_0  searchMode=Binary Search  cacheBpFlag=on  outputFlag=off  IndexDataType=uint32  extrapMode=Linear Extrapolation  rangeErrorMode=None
  AlphaLookup0 : simulink/Lookup Tables/PreLookup Index Search  bpData=alpha_vec_0  searchMode=Binary Search  cacheBpFlag=on  outputFlag=off  IndexDataType=uint32  extrapMode=Linear Extrapolation  rangeErrorMode=None
  Elevator : Subsystem  PropExecContextAcrossSSBoundary=on
  Flap(diff) : Subsystem  PropExecContextAcrossSSBoundary=on
  Flap(neg) : Subsystem  PropExecContextAcrossSSBoundary=on
  Flap(pos) : Subsystem  PropExecContextAcrossSSBoundary=on
  Rudder : Subsystem  PropExecContextAcrossSSBoundary=on
  Sum : Sum  Inputs=++++++  SaturateOnIntegerOverflow=on  InputSameDT=on
  Terminator1 : Terminator
  cl : Outport  InitialOutput=0
  wires:
  AlphaLookup0/1 -> Rudder/1(Alpha), Aileron/1(Alpha)
  (0 to inf) Constants Held fixed for alpha<0/1 -> AlphaLookup0/1
  "Actuator Deflections "/1 -> Aileron/2(Actuators), Elevator/2(Actuators), Rudder/2(Actuators), Flap(pos)/2(Actuators), Flap(neg)/2(Actuators), Flap(diff)/2(Actuators)
  Alpha/1 -> (0 to inf) Constants Held fixed for alpha<0/1, AlphaLookup/1
  Beta/1 -> Terminator1/1
  Aileron/1(delCoeff) -> Sum/1
  Elevator/1(delCoeff) -> Sum/2
  Rudder/1(delCoeff) -> Sum/3
  Flap(pos)/1(delCoeff) -> Sum/4
  Flap(neg)/1(delCoeff) -> Sum/5
  Flap(diff)/1(delCoeff) -> Sum/6
  Sum/1 -> cl/1
  AlphaLookup/1 -> Flap(diff)/1(Alpha), Flap(neg)/1(Alpha), Flap(pos)/1(Alpha), Elevator/1(Alpha)

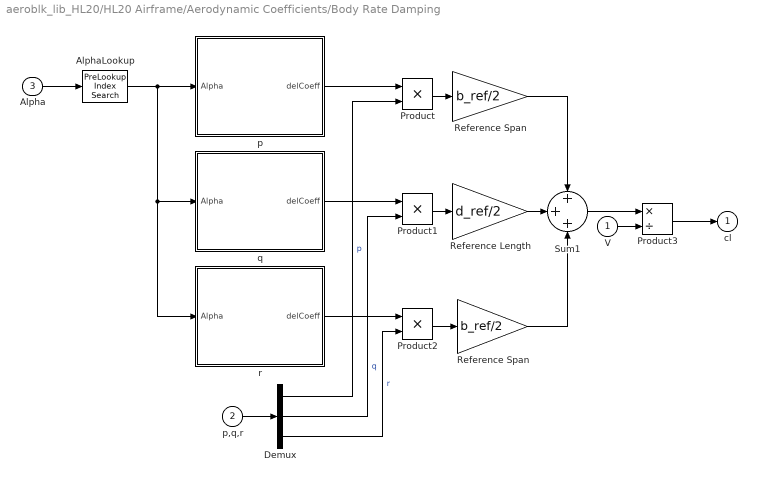
== system aeroblk_lib_HL20/HL20 Airframe/Aerodynamic Coefficients/Body Rate Damping ==
  V : Inport  Port=1  LatchInput=off
  p,q,r : Inport  Port=2  LatchInput=off
  Alpha : Inport  Port=3  LatchInput=off
  AlphaLookup : simulink/Lookup Tables/PreLookup Index Search  bpData=alpha_vec_damping  searchMode=Binary Search  cacheBpFlag=on  outputFlag=off  IndexDataType=uint32  extrapMode=Linear Extrapolation  rangeErrorMode=None
  Demux : Demux  Outputs=3
  Product : Product  SaturateOnIntegerOverflow=on  InputSameDT=on
  Product1 : Product  SaturateOnIntegerOverflow=on  InputSameDT=on
  Product2 : Product  SaturateOnIntegerOverflow=on  InputSameDT=on
  Product3 : Product  Inputs=*/  SaturateOnIntegerOverflow=on  InputSameDT=on
  Reference Length : Gain  Gain=d_ref/2  SaturateOnIntegerOverflow=on
  Reference Span : Gain  Gain=b_ref/2  SaturateOnIntegerOverflow=on
  "Reference Span " : Gain  Gain=b_ref/2  SaturateOnIntegerOverflow=on
  Sum1 : Sum  Inputs=+++  SaturateOnIntegerOverflow=on  InputSameDT=on
  p : Subsystem  PropExecContextAcrossSSBoundary=on
  q : Subsystem  PropExecContextAcrossSSBoundary=on
  r : Subsystem  PropExecContextAcrossSSBoundary=on
  cl : Outport  InitialOutput=0
  wires:
  Alpha/1 -> AlphaLookup/1
  p/1(delCoeff) -> Product/1
  q/1(delCoeff) -> Product1/1
  p,q,r/1 -> Demux/1
  Demux/1 -> Product/2  "p"
  Demux/2 -> Product1/2  "q"
  Demux/3 -> Product2/2  "r"
  Sum1/1 -> Product3/1
  V/1 -> Product3/2
  Product3/1 -> cl/1
  Product1/1 -> Reference Length/1
  Product2/1 -> "Reference Span "/1
  Product/1 -> Reference Span/1
  r/1(delCoeff) -> Product2/1
  AlphaLookup/1 -> r/1(Alpha), q/1(Alpha), p/1(Alpha)
  Reference Length/1 -> Sum1/2
  Reference Span/1 -> Sum1/1
  "Reference Span "/1 -> Sum1/3

== system aeroblk_lib_HL20/HL20 Airframe/Aerodynamic Coefficients/Datum Coefficients ==
  Alpha : Inport  Port=1  LatchInput=off
  Beta : Inport  Port=2  LatchInput=off
  " Cn" : simulink/Lookup Tables/Lookup Table (n-D)  numDimsPopupSelect=2  bp1=alpha_vec_Cn0  bp2=beta_vec_Cn0  bp3=[1:3]  bp4=[1:3]  bpcell={ [1:3], [1:3] }  explicitNumDims=2  searchMode=Binary Search  cacheBpFlag=off  vectorInputFlag=off  tableData=Cn0  interpMethod=Linear  extrapMethod=Linear  rangeErrorMode=None
  Abs : Abs  SaturateOnIntegerOverflow=on
  AlphaLookup : simulink/Lookup Tables/PreLookup Index Search  bpData=alpha_vec_0  searchMode=Binary Search  cacheBpFlag=on  outputFlag=off  IndexDataType=uint32  extrapMode=Linear Extrapolation  rangeErrorMode=None
  BetaLookup : simulink/Lookup Tables/PreLookup Index Search  bpData=beta_vec_0  searchMode=Binary Search  cacheBpFlag=on  outputFlag=off  IndexDataType=uint32  extrapMode=Linear Extrapolation  rangeErrorMode=None
  Cl : Gain  Gain=Clbeta  SaturateOnIntegerOverflow=on
  Cm : simulink/Lookup Tables/Interpolation (n-D) using PreLookup  numDimsPopupSelect=2  explicitNumDims=2  table=Cm0'  interpMethod=Linear  extrapMethod=Linear  rangeErrorMode=None  NumSelectionDims=0
  Cx : simulink/Lookup Tables/Interpolation (n-D) using PreLookup  numDimsPopupSelect=2  explicitNumDims=2  table=CX0'  interpMethod=Linear  extrapMethod=Linear  rangeErrorMode=None  NumSelectionDims=0
  Cy : Gain  Gain=CYbeta  SaturateOnIntegerOverflow=on
  Cz : simulink/Lookup Tables/Interpolation (n-D) using PreLookup  numDimsPopupSelect=2  explicitNumDims=2  table=CZ0'  interpMethod=Linear  extrapMethod=Linear  rangeErrorMode=None  NumSelectionDims=0
  Mux1 : Mux  Inputs=6
  Product : Product  SaturateOnIntegerOverflow=on  InputSameDT=on
  Sign : Signum
  cl : Outport  InitialOutput=0
  wires:
  Sign/1 -> Product/2
  " Cn"/1 -> Product/1
  Product/1 -> Mux1/6
  Abs/1 -> " Cn"/2
  Mux1/1 -> cl/1
  Cx/1 -> Mux1/1
  Cz/1 -> Mux1/3
  Cm/1 -> Mux1/5
  Cy/1 -> Mux1/2
  Cl/1 -> Mux1/4
  Alpha/1 -> AlphaLookup/1, " Cn"/1
  Beta/1 -> BetaLookup/1, Cy/1, Sign/1, Abs/1, Cl/1
  AlphaLookup/1 -> Cx/1, Cm/1, Cz/1
  BetaLookup/1 -> Cz/2, Cm/2, Cx/2

== system aeroblk_lib_HL20/HL20 Airframe/Environment Models/Wind Models ==
  Euler : Inport  Port=1  LatchInput=off
  Ve : Inport  Port=2  LatchInput=off
  Airspeed : Inport  Port=3  LatchInput=off
  Altitude : Inport  Port=4  LatchInput=off
  DCM : Inport  Port=5  LatchInput=off
  Discrete Wind Gust Model - On : aerolibwind2/Discrete Wind Gust Model  units=Metric (MKS)  Gx=on  Gy=on  Gz=on  t_0=20  d_m=[120 120 80]  v_m=[3.5 3.0 3.0]
  Dryden Wind Turbulence Model  (Continuous (+q -r)) : aerolibwind2/Dryden Wind Turbulence Model  (Continuous (+q -r))  units=Metric (MKS)  spec=MIL-F-8785C  model=Continuous Dryden (+q -r)  W20=5  Wdeg=0  TurbProb=10^-2 - Light  L_high=533.4  Wingspan=4  ts=0.1  Seed=[23341 23342 23343 23344]  T_on=on
  Sum : Sum  Inputs=+++  SaturateOnIntegerOverflow=on  InputSameDT=on
  Terminator : Terminator
  Terminator1 : Terminator
  Wind Shear Model : aerolibwind2/Wind Shear Model  units=Metric (MKS)  phase=Category C - Terminal Flight Phase  W_20=1  Wdeg=0
  ug,vg,wg : Outport
  pg,qg,rg : Outport  Port=2
  wires:
  Altitude/1 -> Wind Shear Model/1, Dryden Wind Turbulence Model  (Continuous (+q -r))/1
  Dryden Wind Turbulence Model  (Continuous (+q -r))/2 -> pg,qg,rg/1
  Airspeed/1 -> Discrete Wind Gust Model - On/1, Dryden Wind Turbulence Model  (Continuous (+q -r))/2
  DCM/1 -> Wind Shear Model/2, Dryden Wind Turbulence Model  (Continuous (+q -r))/3
  Sum/1 -> ug,vg,wg/1
  Discrete Wind Gust Model - On/1 -> Sum/3
  Dryden Wind Turbulence Model  (Continuous (+q -r))/1 -> Sum/2
  Wind Shear Model/1 -> Sum/1
  Ve/1 -> Terminator/1
  Euler/1 -> Terminator1/1

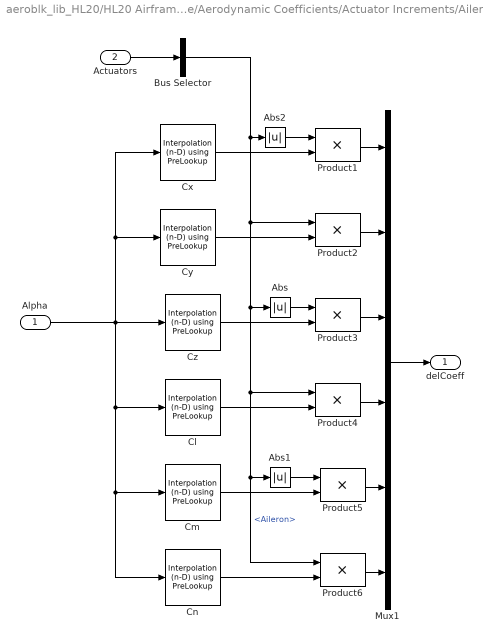
== system aeroblk_lib_HL20/HL20 Airframe/Aerodynamic Coefficients/Actuator Increments/Aileron ==
  Alpha : Inport  Port=1  LatchInput=off
  Actuators : Inport  Port=2  LatchInput=off
  Abs : Abs  SaturateOnIntegerOverflow=on
  Abs1 : Abs  SaturateOnIntegerOverflow=on
  Abs2 : Abs  SaturateOnIntegerOverflow=on
  Bus Selector : BusSelector  DialogController=Simulink.DDGSource_Bus  OutputSignals=Aileron
  Cl : simulink/Lookup Tables/Interpolation (n-D) using PreLookup  numDimsPopupSelect=1  explicitNumDims=2  table=Clda  interpMethod=Linear  extrapMethod=Linear  rangeErrorMode=None  NumSelectionDims=0
  Cm : simulink/Lookup Tables/Interpolation (n-D) using PreLookup  numDimsPopupSelect=1  explicitNumDims=2  table=Cmda  interpMethod=Linear  extrapMethod=Linear  rangeErrorMode=None  NumSelectionDims=0
  Cn : simulink/Lookup Tables/Interpolation (n-D) using PreLookup  numDimsPopupSelect=1  explicitNumDims=2  table=Cnda  interpMethod=Linear  extrapMethod=Linear  rangeErrorMode=None  NumSelectionDims=0
  Cx : simulink/Lookup Tables/Interpolation (n-D) using PreLookup  numDimsPopupSelect=1  explicitNumDims=2  table=CXda  interpMethod=Linear  extrapMethod=Linear  rangeErrorMode=None  NumSelectionDims=0
  Cy : simulink/Lookup Tables/Interpolation (n-D) using PreLookup  numDimsPopupSelect=1  explicitNumDims=2  table=CYda  interpMethod=Linear  extrapMethod=Linear  rangeErrorMode=None  NumSelectionDims=0
  Cz : simulink/Lookup Tables/Interpolation (n-D) using PreLookup  numDimsPopupSelect=1  explicitNumDims=2  table=CZda  interpMethod=Linear  extrapMethod=Linear  rangeErrorMode=None  NumSelectionDims=0
  Mux1 : Mux  Inputs=6
  Product{1..6} (6 alike) : Product  SaturateOnIntegerOverflow=on  InputSameDT=on
  delCoeff : Outport
  wires:
  Alpha/1 -> Cx/1, Cy/1, Cz/1, Cm/1, Cn/1, Cl/1
  Actuators/1 -> Bus Selector/1
  Mux1/1 -> delCoeff/1
  Product1/1 -> Mux1/1
  Cx/1 -> Product1/2
  Product2/1 -> Mux1/2
  Cy/1 -> Product2/2
  Product3/1 -> Mux1/3
  Cz/1 -> Product3/2
  Cl/1 -> Product4/2
  Product4/1 -> Mux1/4
  Cm/1 -> Product5/2
  Product5/1 -> Mux1/5
  Cn/1 -> Product6/2
  Product6/1 -> Mux1/6
  Bus Selector/1 -> Product6/1, Abs1/1, Product4/1, Abs/1, Product2/1, Abs2/1  "<Aileron>"
  Abs/1 -> Product3/1
  Abs1/1 -> Product5/1
  Abs2/1 -> Product1/1

== system aeroblk_lib_HL20/HL20 Airframe/Aerodynamic Coefficients/Actuator Increments/Elevator ==
  Alpha : Inport  Port=1  LatchInput=off
  Actuators : Inport  Port=2  LatchInput=off
  Bus Selector1 : BusSelector  DialogController=Simulink.DDGSource_Bus  OutputSignals=Elevator
  Cm : simulink/Lookup Tables/Interpolation (n-D) using PreLookup  numDimsPopupSelect=1  explicitNumDims=2  table=Cmde  interpMethod=Linear  extrapMethod=Linear  rangeErrorMode=None  NumSelectionDims=0
  Constant1 : Constant  Value=0
  Cx : simulink/Lookup Tables/Interpolation (n-D) using PreLookup  numDimsPopupSelect=1  explicitNumDims=2  table=CXde  interpMethod=Linear  extrapMethod=Linear  rangeErrorMode=None  NumSelectionDims=0
  Cz : simulink/Lookup Tables/Interpolation (n-D) using PreLookup  numDimsPopupSelect=1  explicitNumDims=2  table=CZde  interpMethod=Linear  extrapMethod=Linear  rangeErrorMode=None  NumSelectionDims=0
  Mux1 : Mux  Inputs=6
  Product : Product  SaturateOnIntegerOverflow=on  InputSameDT=on
  delCoeff : Outport
  wires:
  Product/1 -> delCoeff/1
  Mux1/1 -> Product/1
  Alpha/1 -> Cz/1, Cx/1, Cm/1
  Cx/1 -> Mux1/1
  Cz/1 -> Mux1/3
  Cm/1 -> Mux1/5
  Constant1/1 -> Mux1/2, Mux1/4, Mux1/6
  Actuators/1 -> Bus Selector1/1
  Bus Selector1/1 -> Product/2  "<Elevator>"

== system aeroblk_lib_HL20/HL20 Airframe/Aerodynamic Coefficients/Actuator Increments/Flap(diff) ==
  Alpha : Inport  Port=1  LatchInput=off
  Actuators : Inport  Port=2  LatchInput=off
  Abs2 : Abs  SaturateOnIntegerOverflow=on
  Bus Selector : BusSelector  DialogController=Simulink.DDGSource_Bus  OutputSignals=Flap(diff)
  Cl : simulink/Lookup Tables/Interpolation (n-D) using PreLookup  numDimsPopupSelect=1  explicitNumDims=2  table=Clddf  interpMethod=Linear  extrapMethod=Linear  rangeErrorMode=None  NumSelectionDims=0
  Cn : simulink/Lookup Tables/Interpolation (n-D) using PreLookup  numDimsPopupSelect=1  explicitNumDims=2  table=Cnddf  interpMethod=Linear  extrapMethod=Linear  rangeErrorMode=None  NumSelectionDims=0
  Constant1 : Constant  Value=0
  Cx : simulink/Lookup Tables/Interpolation (n-D) using PreLookup  numDimsPopupSelect=1  explicitNumDims=2  table=CXddf  interpMethod=Linear  extrapMethod=Linear  rangeErrorMode=None  NumSelectionDims=0
  Cy : simulink/Lookup Tables/Interpolation (n-D) using PreLookup  numDimsPopupSelect=1  explicitNumDims=2  table=CYddf  interpMethod=Linear  extrapMethod=Linear  rangeErrorMode=None  NumSelectionDims=0
  Mux1 : Mux  Inputs=6
  Product{,1..3} (4 alike) : Product  SaturateOnIntegerOverflow=on  InputSameDT=on
  delCoeff : Outport
  wires:
  Mux1/1 -> delCoeff/1
  Alpha/1 -> Cl/1, Cn/1, Cy/1, Cx/1
  Actuators/1 -> Bus Selector/1
  Product/1 -> Mux1/1
  Cx/1 -> Product/2
  Bus Selector/1 -> Product3/1, Product2/1, Product1/1, Abs2/1  "<Flap(diff)>"
  Product1/1 -> Mux1/2
  Product2/1 -> Mux1/4
  Cl/1 -> Product2/2
  Cy/1 -> Product1/2
  Product3/1 -> Mux1/6
  Cn/1 -> Product3/2
  Abs2/1 -> Product/1
  Constant1/1 -> Mux1/3, Mux1/5

== system aeroblk_lib_HL20/HL20 Airframe/Aerodynamic Coefficients/Actuator Increments/Flap(neg) ==
  Alpha : Inport  Port=1  LatchInput=off
  Actuators : Inport  Port=2  LatchInput=off
  Bus Selector : BusSelector  DialogController=Simulink.DDGSource_Bus  OutputSignals=Flap(neg)
  Cm : simulink/Lookup Tables/Interpolation (n-D) using PreLookup  numDimsPopupSelect=1  explicitNumDims=2  table=Cmdfn  interpMethod=Linear  extrapMethod=Linear  rangeErrorMode=None  NumSelectionDims=0
  Constant1 : Constant  Value=0
  Constant2 : Constant  Value=0
  Constant3 : Constant  Value=0
  Cx : simulink/Lookup Tables/Interpolation (n-D) using PreLookup  numDimsPopupSelect=1  explicitNumDims=2  table=CXdfn  interpMethod=Linear  extrapMethod=Linear  rangeErrorMode=None  NumSelectionDims=0
  Cz : simulink/Lookup Tables/Interpolation (n-D) using PreLookup  numDimsPopupSelect=1  explicitNumDims=2  table=CZdfn  interpMethod=Linear  extrapMethod=Linear  rangeErrorMode=None  NumSelectionDims=0
  Mux1 : Mux  Inputs=6
  Product : Product  SaturateOnIntegerOverflow=on  InputSameDT=on
  delCoeff : Outport
  wires:
  Cm/1 -> Mux1/5
  Cz/1 -> Mux1/3
  Cx/1 -> Mux1/1
  Alpha/1 -> Cz/1, Cm/1, Cx/1
  Mux1/1 -> Product/1
  Product/1 -> delCoeff/1
  Actuators/1 -> Bus Selector/1
  Constant1/1 -> Mux1/2
  Constant2/1 -> Mux1/4
  Constant3/1 -> Mux1/6
  Bus Selector/1 -> Product/2  "<Flap(neg)>"

== system aeroblk_lib_HL20/HL20 Airframe/Aerodynamic Coefficients/Actuator Increments/Flap(pos) ==
  Alpha : Inport  Port=1  LatchInput=off
  Actuators : Inport  Port=2  LatchInput=off
  Bus Selector : BusSelector  DialogController=Simulink.DDGSource_Bus  OutputSignals=Flap(pos)
  Cm : simulink/Lookup Tables/Interpolation (n-D) using PreLookup  numDimsPopupSelect=1  explicitNumDims=2  table=Cmdfp  interpMethod=Linear  extrapMethod=Linear  rangeErrorMode=None  NumSelectionDims=0
  Constant1 : Constant  Value=0
  Constant2 : Constant  Value=0
  Constant3 : Constant  Value=0
  Cx : simulink/Lookup Tables/Interpolation (n-D) using PreLookup  numDimsPopupSelect=1  explicitNumDims=2  table=CXdfp  interpMethod=Linear  extrapMethod=Linear  rangeErrorMode=None  NumSelectionDims=0
  Cz : simulink/Lookup Tables/Interpolation (n-D) using PreLookup  numDimsPopupSelect=1  explicitNumDims=2  table=CZdfp  interpMethod=Linear  extrapMethod=Linear  rangeErrorMode=None  NumSelectionDims=0
  Mux1 : Mux  Inputs=6
  Product : Product  SaturateOnIntegerOverflow=on  InputSameDT=on
  delCoeff : Outport
  wires:
  Product/1 -> delCoeff/1
  Mux1/1 -> Product/1
  Alpha/1 -> Cz/1, Cm/1, Cx/1
  Cx/1 -> Mux1/1
  Cz/1 -> Mux1/3
  Cm/1 -> Mux1/5
  Constant1/1 -> Mux1/2
  Constant2/1 -> Mux1/4
  Constant3/1 -> Mux1/6
  Actuators/1 -> Bus Selector/1
  Bus Selector/1 -> Product/2  "<Flap(pos)>"

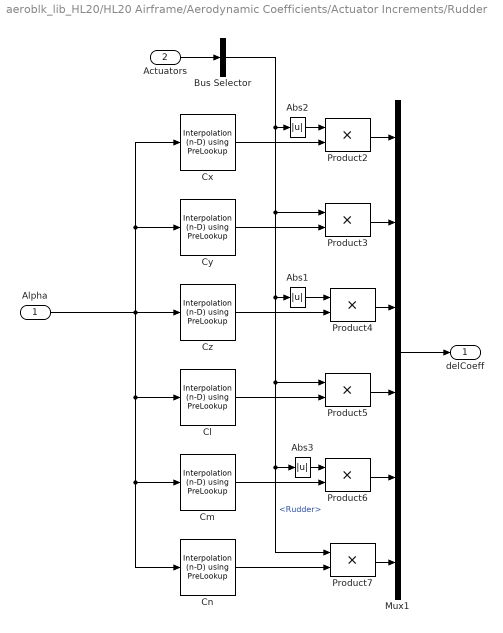
== system aeroblk_lib_HL20/HL20 Airframe/Aerodynamic Coefficients/Actuator Increments/Rudder ==
  Alpha : Inport  Port=1  LatchInput=off
  Actuators : Inport  Port=2  LatchInput=off
  Abs1 : Abs  SaturateOnIntegerOverflow=on
  Abs2 : Abs  SaturateOnIntegerOverflow=on
  Abs3 : Abs  SaturateOnIntegerOverflow=on
  Bus Selector : BusSelector  DialogController=Simulink.DDGSource_Bus  OutputSignals=Rudder
  Cl : simulink/Lookup Tables/Interpolation (n-D) using PreLookup  numDimsPopupSelect=1  explicitNumDims=2  table=Cldr  interpMethod=Linear  extrapMethod=Linear  rangeErrorMode=None  NumSelectionDims=0
  Cm : simulink/Lookup Tables/Interpolation (n-D) using PreLookup  numDimsPopupSelect=1  explicitNumDims=2  table=Cmdr  interpMethod=Linear  extrapMethod=Linear  rangeErrorMode=None  NumSelectionDims=0
  Cn : simulink/Lookup Tables/Interpolation (n-D) using PreLookup  numDimsPopupSelect=1  explicitNumDims=2  table=Cndr  interpMethod=Linear  extrapMethod=Linear  rangeErrorMode=None  NumSelectionDims=0
  Cx : simulink/Lookup Tables/Interpolation (n-D) using PreLookup  numDimsPopupSelect=1  explicitNumDims=2  table=CXdr  interpMethod=Linear  extrapMethod=Linear  rangeErrorMode=None  NumSelectionDims=0
  Cy : simulink/Lookup Tables/Interpolation (n-D) using PreLookup  numDimsPopupSelect=1  explicitNumDims=2  table=CYdr  interpMethod=Linear  extrapMethod=Linear  rangeErrorMode=None  NumSelectionDims=0
  Cz : simulink/Lookup Tables/Interpolation (n-D) using PreLookup  numDimsPopupSelect=1  explicitNumDims=2  table=CZdr  interpMethod=Linear  extrapMethod=Linear  rangeErrorMode=None  NumSelectionDims=0
  Mux1 : Mux  Inputs=6
  Product{2..7} (6 alike) : Product  SaturateOnIntegerOverflow=on  InputSameDT=on
  delCoeff : Outport
  wires:
  Alpha/1 -> Cx/1, Cy/1, Cz/1, Cl/1, Cm/1, Cn/1
  Mux1/1 -> delCoeff/1
  Actuators/1 -> Bus Selector/1
  Cx/1 -> Product2/2
  Product2/1 -> Mux1/1
  Cy/1 -> Product3/2
  Product3/1 -> Mux1/2
  Cz/1 -> Product4/2
  Product4/1 -> Mux1/3
  Cl/1 -> Product5/2
  Product5/1 -> Mux1/4
  Cm/1 -> Product6/2
  Product6/1 -> Mux1/5
  Cn/1 -> Product7/2
  Product7/1 -> Mux1/6
  Bus Selector/1 -> Product3/1, Product5/1, Product7/1, Abs3/1, Abs1/1, Abs2/1  "<Rudder>"
  Abs2/1 -> Product2/1
  Abs1/1 -> Product4/1
  Abs3/1 -> Product6/1

== system aeroblk_lib_HL20/HL20 Airframe/Aerodynamic Coefficients/Body Rate Damping/p ==
  Alpha : Inport  Port=1  LatchInput=off
  Cl : simulink/Lookup Tables/Interpolation (n-D) using PreLookup  numDimsPopupSelect=1  explicitNumDims=2  table=Clp  interpMethod=Linear  extrapMethod=Linear  rangeErrorMode=None  NumSelectionDims=0
  Cn : simulink/Lookup Tables/Interpolation (n-D) using PreLookup  numDimsPopupSelect=1  explicitNumDims=2  table=Cnp  interpMethod=Linear  extrapMethod=Linear  rangeErrorMode=None  NumSelectionDims=0
  Constant1 : Constant  Value=0
  Mux1 : Mux  Inputs=6
  delCoeff : Outport
  wires:
  Mux1/1 -> delCoeff/1
  Constant1/1 -> Mux1/1, Mux1/5, Mux1/3, Mux1/2  "Cxp"
  Cn/1 -> Mux1/6
  Cl/1 -> Mux1/4  "Cl"
  Alpha/1 -> Cl/1, Cn/1
